simulink model "example_embeddedMatlabBlock"  (R2012b)
settings: Solver=ode45  StartTime=0.0  StopTime=10.0  RelTol=1e-3
settings Model: Creator=j.bolting  LastModifiedBy=j.bolting

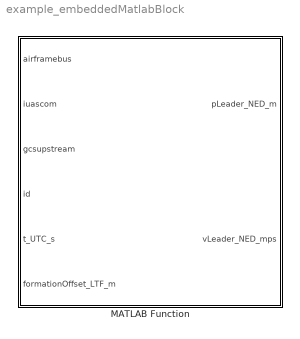
== system example_embeddedMatlabBlock ==
  MATLAB Function : MATLAB Function  TreatAsAtomicUnit=on

== matlab function example_embeddedMatlabBlock/MATLAB Function ==
  data: airframebus input; iuascom input; gcsupstream input; id input; pLeader_NED_m output; vLeader_NED_mps output; t_UTC_s input; formationOffset_LTF_m input
function [pLeader_NED_m,vLeader_NED_mps] = doItNow(airframebus, iuascom, gcsupstream, id, t_UTC_s, formationOffset_LTF_m)
%#codegen
% Holds the current trajectory to be followed:
persistent traj;
% Holds the UTC start time of the current trajectory:
persistent traj_t0_UTC_s;
% Holds the trajectory ground speed:
traj_v_mps = 15;

% The following functions use language elements that are not supported for
% code generation and have to be replaced for implementation on the
% autopilot:
coder.extrinsic('trajectory_build');
coder.extrinsic('trajectory_smooth');
coder.extrinsic('trajectory_concatenateWaypoint');
coder.extrinsic('trajectory_getAirborne');
coder.extrinsic('trajectory_get');
coder.extrinsic('trajectory_display');
coder.extrinsic('trajectory_concatenateLoiterPattern');

% Strategy:
% - Compute trajectory that catches the virtual leader's holding trajectory
% - The first lag of the trajectory leads to the formation approach flight
%   level of this UAS.
[pNow_leader_NED_m, vNow_leader_NED_mps] = getLeaderState(t_UTC_s, gcsupstream);

% Check whether we are close enough to the virtual leader to follow it (into the dark)
% without any trajectory replanning:
% Commanded position in formation:
offset_NED_m = ltf2ned(formationOffset_LTF_m, vNow_leader_NED_mps);
pc_NED_m = pNow_leader_NED_m + offset_NED_m;
if norm(pc_NED_m - airframebus.Kinematics.Position.P_NED_m) < 5
    % Transform formation offset from LT frame to NED frame:
    pLeader_NED_m = pc_NED_m;
    vLeader_NED_mps = vNow_leader_NED_mps;
else
    if isempty(traj)
    % The flight level is id * altitudeStep above the leader's altitude:
    pLeader_NED_m = pNow_leader_NED_m;
    vLeader_NED_mps = vNow_leader_NED_mps;
    dAlt = 5;
    fl = pLeader_NED_m(3) - dAlt * id;
    
    % Generate transition trajectory to join leader on its holding pattern:
    % Generate holding pattern:
    gamma = deg2rad(20);
    % TODO Does not take into account wind.
    v = norm(vLeader_NED_mps);
    % Climb to flight level, keeping the current flight path angle:
    wp1 = airframebus.Kinematics.Position.P_NED_m;
    traj = trajectory_build(wp1);
    initialFlightPath = fflib_normalize([airframebus.Kinematics.Velocity.Vground_NED_mps(1:2); 0]);
    orthogonalToFlightpath = fflib_normalize(cross([0 0 1]', initialFlightPath));
    initialFlightPath = fflib_normalize([initialFlightPath(1:2); -tan(gamma)]);
    lengthOfFirstLag = (fl - wp1(3)) / initialFlightPath(3);
    % Waypoint increments:
    dwp2 = lengthOfFirstLag * initialFlightPath;
    dwp3 = 200 * fflib_normalize([initialFlightPath(1:2); 0]);
    dwp4 = 300 * orthogonalToFlightpath;
    traj = trajectory_concatenateWaypoint(dwp2, traj);
    traj = trajectory_concatenateWaypoint(dwp3, traj);
    traj = trajectory_concatenateWaypoint(dwp4, traj);
    traj = trajectory_concatenateLoiterPattern(300, traj);
    
    traj = trajectory_smooth(traj, 0.01);
    traj = trajectory_getAirborne(traj);
    
%         plotoptions.controlpointsvisible = false;
%         plotoptions.waypointsvisible = true;
%         plotoptions.discretepointsvisible = true;
%         trajectory_display(traj, plotoptions);
    
    traj_t0_UTC_s = t_UTC_s;
end
    % If still transitioning, compute current position of local leader on
    % current trajectory:
    s = traj_v_mps * (t_UTC_s - traj_t0_UTC_s);
    [p, dpds] = trajectory_get(traj, s);
    
    pLeader_NED_m = p;
    vLeader_NED_mps = dpds * traj_v_mps;
end

end

function p_NED_m = ltf2ned(p_LTF_m, vLeader_NED_mps)
coder.extrinsic('angle2dcm');

chi = atan2(vLeader_NED_mps(2), vLeader_NED_mps(1));
% Rotate:
p_NED_m = zeros(3,1);
p_NED_m = angle2dcm(-chi, 0, 0, 'ZXY') * p_LTF_m;
end

function [p, v] = getLeaderState(t, gcsupstream)
v = zeros(3,1);
p = zeros(3,1);

r0 = gcsupstream.vlMergingpattern_p0_NED_m ...
    - gcsupstream.vlMergingpattern_center_NED_m;
chiDot =  gcsupstream.vlMergingpattern_v_NED_mps / norm(r0);
delta_t = t - gcsupstream.vlMergingpattern_t0_UTC_s;
delta_chi = delta_t * chiDot;
DCM_2D = [cos(delta_chi) -sin(delta_chi);
    sin(delta_chi) cos(delta_chi)];
r2D = DCM_2D * r0(1:2);
r = [r2D; r0(3)];
p = gcsupstream.vlMergingpattern_center_NED_m + r;

v = cross([0 0 1]', r);
v = v/norm(v);
v = gcsupstream.vlMergingpattern_v_NED_mps * v;
end
